simulink subsystem "ModeController"  (R2022a)
settings: Solver=VariableStepAuto  StartTime=0.0  StopTime=10.0  RelTol=1e-3
undefined symbols (not defined in the file): MODE
libraries: simulink x4
settings Model: Creator=bkfre  LastModifiedBy=bkfre

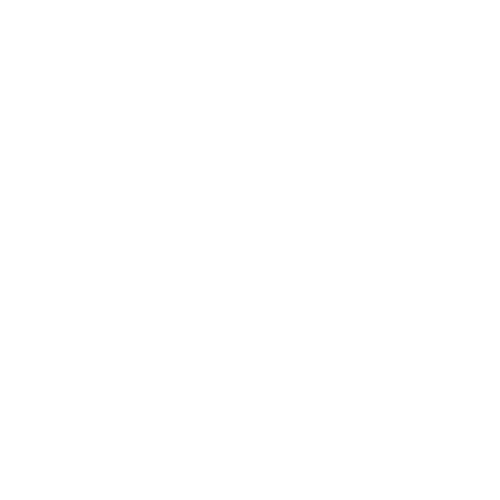
[thumbnail: Simulink's stored preview of the top-level diagram]
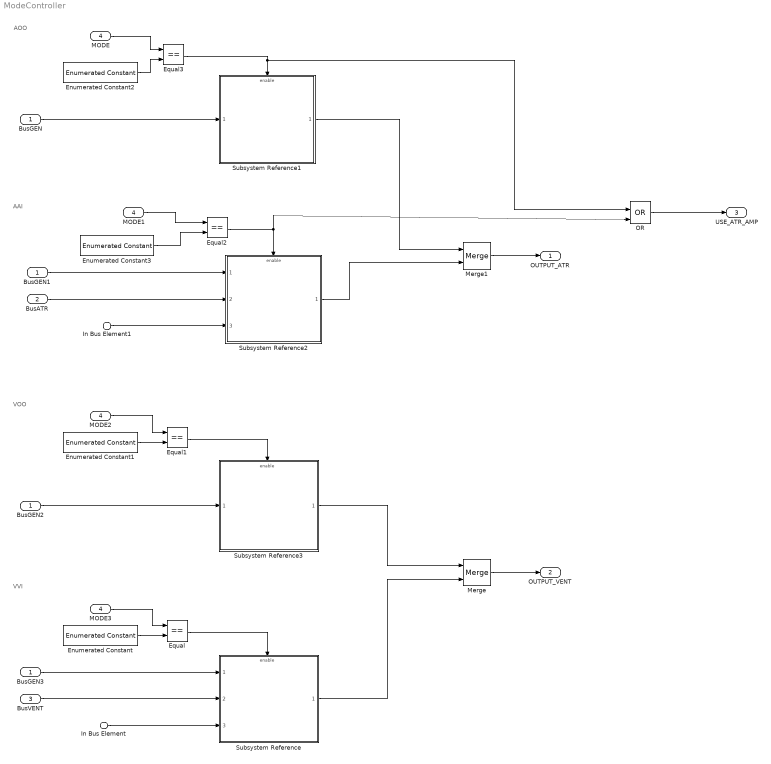
== system ModeController ==
  note: VVI
  note: VOO
  note: AOO
  note: AAI
  BusGEN : Inport  OutDataTypeStr=Bus: BusGEN
  BusATR : Inport  Port=2  OutDataTypeStr=Bus: BusSPECIFIC
  BusVENT : Inport  Port=3  OutDataTypeStr=Bus: BusSPECIFIC
  MODE : Inport  Port=4
  In Bus Element1 : Inport  Port=5  PortName=BusMEASURED  Element=R_WAVE
  In Bus Element : Inport  Port=5  PortName=BusMEASURED  Element=P_WAVE
  BusGEN1 : InportShadow  OutDataTypeStr=Bus: BusGEN
  BusGEN2 : InportShadow  OutDataTypeStr=Bus: BusGEN
  BusGEN3 : InportShadow  OutDataTypeStr=Bus: BusGEN
  Enumerated Constant : simulink/Sources/Enumerated Constant  OutDataTypeStr=Enum: MODE  Value=MODE.VVI  SampleTime=inf
  Enumerated Constant1 : simulink/Sources/Enumerated Constant  OutDataTypeStr=Enum: MODE  Value=MODE.VOO  SampleTime=inf
  Enumerated Constant2 : simulink/Sources/Enumerated Constant  OutDataTypeStr=Enum: MODE  Value=MODE.AOO  SampleTime=inf
  Enumerated Constant3 : simulink/Sources/Enumerated Constant  OutDataTypeStr=Enum: MODE  Value=MODE.AAI  SampleTime=inf
  Equal{,1..3} (4 alike) : RelationalOperator  Operator===  RndMeth=Simplest  InputSameDT=off
  MODE1 : InportShadow  Port=4
  MODE2 : InportShadow  Port=4
  MODE3 : InportShadow  Port=4
  Merge : Merge
  Merge1 : Merge
  OR : Logic  Operator=OR  IconShape=distinctive  AllPortsSameDT=off  OutDataTypeStr=boolean
  Subsystem Reference : Subsystem  ReferencedSubsystem=mode_xxI
  Subsystem Reference1 : Subsystem  ReferencedSubsystem=mode_xOO
  Subsystem Reference2 : Subsystem  ReferencedSubsystem=mode_xxI
  Subsystem Reference3 : Subsystem  ReferencedSubsystem=mode_xOO
  OUTPUT_ATR : Outport
  OUTPUT_VENT : Outport  Port=2
  USE_ATR_AMP : Outport  Port=3
  wires:
  Subsystem Reference3/1 -> Merge/1
  Subsystem Reference/1 -> Merge/2
  Merge/1 -> OUTPUT_VENT/1
  Subsystem Reference1/1 -> Merge1/1
  Subsystem Reference2/1 -> Merge1/2
  Merge1/1 -> OUTPUT_ATR/1
  Enumerated Constant/1 -> Equal/2
  Equal/1 -> Subsystem Reference/Enable
  Enumerated Constant2/1 -> Equal3/2
  Equal3/1 -> Subsystem Reference1/Enable, OR/1
  Equal2/1 -> OR/2, Subsystem Reference2/Enable
  Enumerated Constant3/1 -> Equal2/2
  Equal1/1 -> Subsystem Reference3/Enable
  Enumerated Constant1/1 -> Equal1/2
  MODE/1 -> Equal3/1
  MODE1/1 -> Equal2/1
  MODE2/1 -> Equal1/1
  MODE3/1 -> Equal/1
  BusGEN/1 -> Subsystem Reference1/1
  BusGEN1/1 -> Subsystem Reference2/1
  BusGEN2/1 -> Subsystem Reference3/1
  BusGEN3/1 -> Subsystem Reference/1
  BusATR/1 -> Subsystem Reference2/2
  BusVENT/1 -> Subsystem Reference/2
  OR/1 -> USE_ATR_AMP/1
  In Bus Element/1 -> Subsystem Reference/3
  In Bus Element1/1 -> Subsystem Reference2/3
